simulink model "CM320A_Adc1CfgAndUse"  (R2013b)
settings: Solver=FixedStepDiscrete  SolverMode=SingleTasking  StartTime=0.0  StopTime=1  FixedStep=0.002  RelTol=1e-3
values from neighbouring files (symbols this model uses):
  ADC0CFGANDUSE_DIAGCSCANGROUPMAX_CNT_U08 = DataDict.Constant    [CM320A_Adc1CfgAndUse_DataDict.m]
  ADC0CFGANDUSE_DIAGCSCANGROUPMIN_CNT_U08 = DataDict.Constant    [CM320A_Adc1CfgAndUse_DataDict.m]
undefined symbols (not defined in the file or in its folder): sigbuilder_block
libraries: simulink x3
settings Model: Creator=nz3zln  LastModifiedBy=wzvp6q
settings SolverCC: AutoInsertRateTranBlk=on  InsertRTBMode=Always
settings DataIOCC: LimitDataPoints=off  SaveFormat=Structure  ReturnWorkspaceOutputs=on
settings OptimizationCC: BlockReduction=off  InlineParams=on  ZeroExternalMemoryAtStartup=off  ZeroInternalMemoryAtStartup=off  OptimizeModelRefInitCode=on  LifeSpan=1
settings DebuggingCC: SignalInfNanChecking=error  SignalRangeChecking=warning  UnderspecifiedInitializationDetection=Simplified  SolverPrmCheckMsg=error  DiscreteInheritContinuousMsg=error  SingleTaskRateTransMsg=error  TasksWithSamePriorityMsg=error  SigSpecEnsureSampleTimeMsg=error  CheckMatrixSingularityMsg=error  ParameterUnderflowMsg=error  ParameterPrecisionLossMsg=error  ParameterTunabilityLossMsg=error  FixptConstUnderflowMsg=warning  FixptConstOverflowMsg=warning  VectorMatrixConversionMsg=error  SignalLabelMismatchMsg=error  UnconnectedInputMsg=error  UnconnectedOutputMsg=error  UnconnectedLineMsg=error  SFcnCompatibilityMsg=error  UniqueDataStoreMsg=warning  BusObjectLabelMismatch=error  RootOutportRequireBusObject=error  AssertControl=DisableAll  ModelReferenceIOMsg=error  ModelReferenceVersionMismatchMessage=warning  ModelReferenceIOMismatchMessage=error  ModelReferenceCSMismatchMessage=warning  ModelReferenceDataLoggingMessage=error  StateNameClashWarn=warning  StrictBusMsg=ErrorOnBusTreatedAsVector  NonBusSignalsTreatedAsBus=error  SFUnexpectedBacktrackingDiag=error  SFInvalidInputDataAccessInChartInitDiag=error  SFNoUnconditionalDefaultTransitionDiag=error  SFTransitionOutsideNaturalParentDiag=error  SFUnconditionalTransitionShadowingDiag=error  SFUndirectedBroadcastEventsDiag=error
settings ModelReferenceCC: ModelReferenceNumInstancesAllowed=Single
settings RTWCC: SystemTargetFile=autosar.tlc  GenCodeOnly=on  TemplateMakefile=ert_default_tmf  Description=AUTOSAR  GenerateReport=on  ProcessScript=autosar_make_rtw_hook  LaunchReport=on
settings CodeAppCC: GenerateComments=off  IgnoreCustomStorageClasses=off  CustomSymbolStrType=$N$R$M  CustomSymbolStrBlkIO=$N$M  SimulinkBlockComments=off
settings STFCustomTargetCC: ParMdlRefBuildCompliant=on  CompOptLevelCompliant=on  IncludeMdlTerminateFcn=off  CombineOutputUpdateFcns=on  SuppressErrorStatus=on  ERTFirstTimeCompliant=on  ERTCustomFileBanners=on  SupportNonFinite=off  SupportComplex=off  SupportContinuousTime=off  SupportNonInlinedSFcns=off  MATLABClassNameForMDSCustomization=Simulink.SoftwareTarget.ERTCustomization  AutosarCompliant=on  GRTInterface=off  SystemTargetFile=autosar.tlc
settings ERTTargetCC: CodeReplacementLibrary=ANSI_C  ConcurrentExecutionCompliant=off  IncludeMdlTerminateFcn=off  SuppressErrorStatus=on  SupportNonFinite=off  SupportComplex=off  ModelStepFunctionPrototypeControlCompliant=off  CPPClassGenCompliant=off  AutosarCompliant=on  InlinedParameterPlacement=NonHierarchical  ERTCustomFileTemplate=example_file_process.tlc  EnableUserReplacementTypes=on

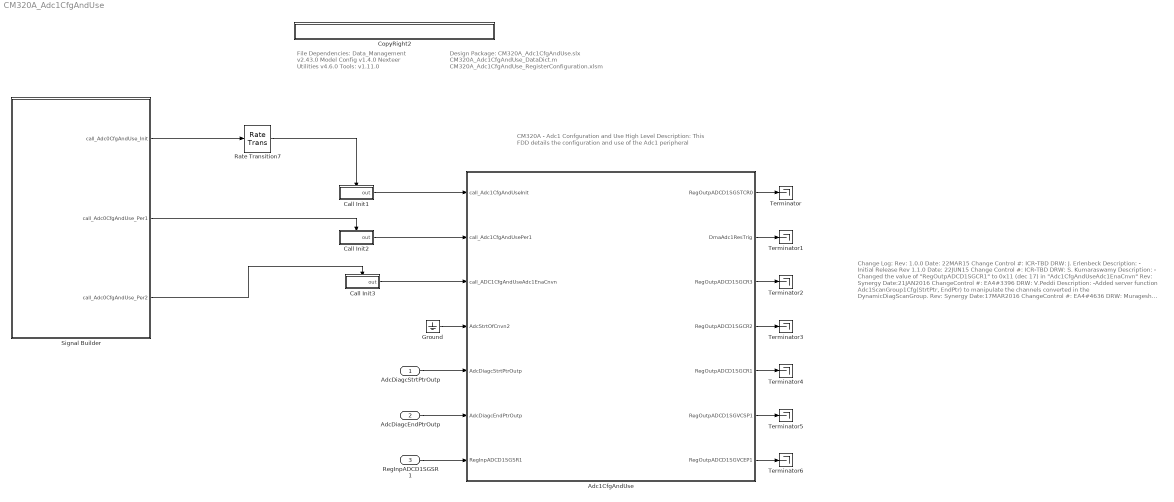
== system CM320A_Adc1CfgAndUse ==
  note: CM320A - Adc1 Confguration and Use
      |
      | High Level Description:
      | This FDD details the configuration and use of the Adc1 peripheral
  note: Change Log:
      |
      | Rev: 1.0.0
      | Date: 22MAR15
      | Change Control #: ICR-TBD
      | DRW: J. Erlenbeck
      | Description:
      | - Initial Release
      |
      | Rev 1.1.0
      | Date: 22JUN15
      | Change Control #: ICR-TBD
      | DRW: S. Kumaraswamy
      | Description:
      | - Changed the value of "RegOutpADCD1SGCR1" to 0x11 (dec 17) in "Adc1CfgAndUseAdc1EnaCnvn"
      |
      | Rev: Synergy
      | Date:21JAN2016
      | ChangeControl #: EA4#3396
      | DRW: V.Peddi
      | Description:
      | -Added server function Adc1ScanGroup1Cfg(StrtPtr, EndPtr)
      |  to manipulate the channels converted in the DynamicDiagScanGroup.
      |
      |
      | Rev: Synergy
      | Date:17MAR2016
      | ChangeControl #: EA4#4636
      | DRW: Muragesh Asundi/Lalkrishna Pandey (KPIT)
      | Description:
      | -As per anomaly CR EA4#3742, following changes are made,
      | -  Register names ADCD0SGVCEP1 and ADCD0SGVCSP1 corrected to
      | ADCD1SGVCEP1 and ADCD1SGVCSP1 respectively.
      | - All the constants and configParam properties are updated to 'Global'.
      |
      |
      | Rev 2.2.0
      | Date: 07JUN16
      | Change Control #: WCR EA4#5947
      | DRW: G. McCann
      | Description:
      | - Remove server function Adc1CfgAndUseAdc1ScanGroup1Cfg and
      |   replace with Adc1CfgAndUsePer2
      | - Make StrtPtr and EndPtr update dependent on a change in inputs and
      |   A/D converter idle state
      |
      |
      | Rev 2.3.0
      | Date: 28JUL16
      | Change Control #: WCR EA4#7446
      | DRW: G. McCann
      | Description:
      | - Initialize Adc1DiagcStrtPtr and Adc1DiagcEndPtr in Adc1CfgAndUseInit1
      | - Updated CM320A_Adc1CfgAndUse_RegisterConfiguration.xlsm to use ADCD1SGCR1 to trigger DMA
      |   instead of ADCD1SGCR3 to trigger DMA.
  note: File Dependencies:
      | Data_Management v2.43.0
      | Model Config v1.4.0
      | Nexteer Utilities v4.6.0
      | Tools: v1.11.0
  note: Design Package:
      | CM320A_Adc1CfgAndUse.slx
      | CM320A_Adc1CfgAndUse_DataDict.m
      | CM320A_Adc1CfgAndUse_RegisterConfiguration.xlsm
  AdcDiagcStrtPtrOutp : Inport
  AdcDiagcEndPtrOutp : Inport  Port=2
  RegInpADCD1SGSR1 : Inport  RequirementInfo={} %GIDa_1454e784_31d7_4f3c_b38c_eefbf3be6ffb  Port=3
  Adc1CfgAndUse : Subsystem
  Call Init1 : Subsystem  TreatAsAtomicUnit=on
  Call Init2 : Subsystem  TreatAsAtomicUnit=on
  Call Init3 : Subsystem  TreatAsAtomicUnit=on
  CopyRight2 : Subsystem  Description=|  mask(Copyright Information){none=on}
      | Copyright info block.                                               
      |                                                                     
      | Place copyright information at the top of every subsystem in design.
      mask prompts: none "No parameters"
      mask help: Place copyright information at the top of every subsystem in design.
      mask Display:
      | NxtrConf = 'Nexteer Confidential';
      | 
      | sys = bdroot; %handle for the current model ("system")
      | first = get_param(sys,'Created');
      | first = first(end-3:end);  %year is last four digits
      | 
      | last = get_param(sys,'LastModifiedDate');
      | if isempty(last)
      |     last = datestr(now,'yyyy');
      | else
      |     last = last(end-3:end);
      | end
      | 
      | if strcmp(first,last)
      |     fprintf('%s -- Copyright %s Nexteer',NxtrConf,first)
      | else
      |     fprintf('%s -- %s%s- %s Nexteer',NxtrConf,char(169),first,last)
      | end
  Ground : Ground
  Rate Transition7 : RateTransition
  Signal Builder : Subsystem  Tag=STV Subsys  RequirementInfo={} %GIDa_2822100e_29fa_4197_9ccc_01864625f252  LoadFcn=sigbuilder_block('load');  StartFcn=sigbuilder_block('start');  StopFcn=sigbuilder_block('stop');  ClipboardFcn=sigbuilder_block('clipboard');  mask(Sigbuilder block){}
      mask help: Simulink:masks:SigbuilderBlock_MD
      mask init:
      | if ~strcmp(get_param(bdroot(gcbh),'SimulationStatus'),'stopped') tuvar = sigbuilder_block('maskInit'); end
      settings: CopyFcn=sigbuilder_block('copy');  DeleteFcn=sigbuilder_block('delete');  ModelCloseFcn=sigbuilder_block('modelClose');  PreSaveFcn=sigbuilder_block('preSave');  PauseFcn=sigbuilder_block('pause');  ContinueFcn=sigbuilder_block('continue');  NameChangeFcn=sigbuilder_block('namechange');  OpenFcn=sigbuilder_block('open',[0 127.5 768 484.5 ]);  CloseFcn=sigbuilder_block('close');
      mask Display: plot(0, 0, 100, 100,[2, 2, 32, 32, 2], [68, 8, 8, 68, 68],[32, 2], [38, 38], [32, 19, 2],[53, 60, 44], [32, 17, 17, 2],[16, 16, 31, 31]);txt = getActiveGroup(gcbh);text(2, 100, txt,'verticalAlignment', 'top');
  Terminator{,1..6} (7 alike) : Terminator
  wires:
  Signal Builder/1(call_Adc0CfgAndUse_Init) -> Rate Transition7/1
  Call Init1/1(out) -> Adc1CfgAndUse/1(call_Adc1CfgAndUseInit)
  Rate Transition7/1 -> Call Init1/Enable
  Signal Builder/2(call_Adc0CfgAndUse_Per1) -> Call Init2/Enable
  Signal Builder/3(call_Adc0CfgAndUse_Per2) -> Call Init3/Enable
  Call Init2/1(out) -> Adc1CfgAndUse/2(call_Adc1CfgAndUsePer1)
  Call Init3/1(out) -> Adc1CfgAndUse/3(call_ADC1CfgAndUseAdc1EnaCnvn)
  AdcDiagcStrtPtrOutp/1 -> Adc1CfgAndUse/5(AdcDiagcStrtPtrOutp)
  AdcDiagcEndPtrOutp/1 -> Adc1CfgAndUse/6(AdcDiagcEndPtrOutp)
  RegInpADCD1SGSR1/1 -> Adc1CfgAndUse/7(RegInpADCD1SGSR1)
  Ground/1 -> Adc1CfgAndUse/4(AdcStrtOfCnvn2)
  Adc1CfgAndUse/1(RegOutpADCD1SGSTCR0) -> Terminator/1
  Adc1CfgAndUse/2(DmaAdc1ResTrig) -> Terminator1/1
  Adc1CfgAndUse/3(RegOutpADCD1SGCR3) -> Terminator2/1
  Adc1CfgAndUse/4(RegOutpADCD1SGCR2) -> Terminator3/1
  Adc1CfgAndUse/5(RegOutpADCD1SGCR1) -> Terminator4/1
  Adc1CfgAndUse/6(RegOutpADCD1SGVCSP1) -> Terminator5/1
  Adc1CfgAndUse/7(RegOutpADCD1SGVCEP1) -> Terminator6/1

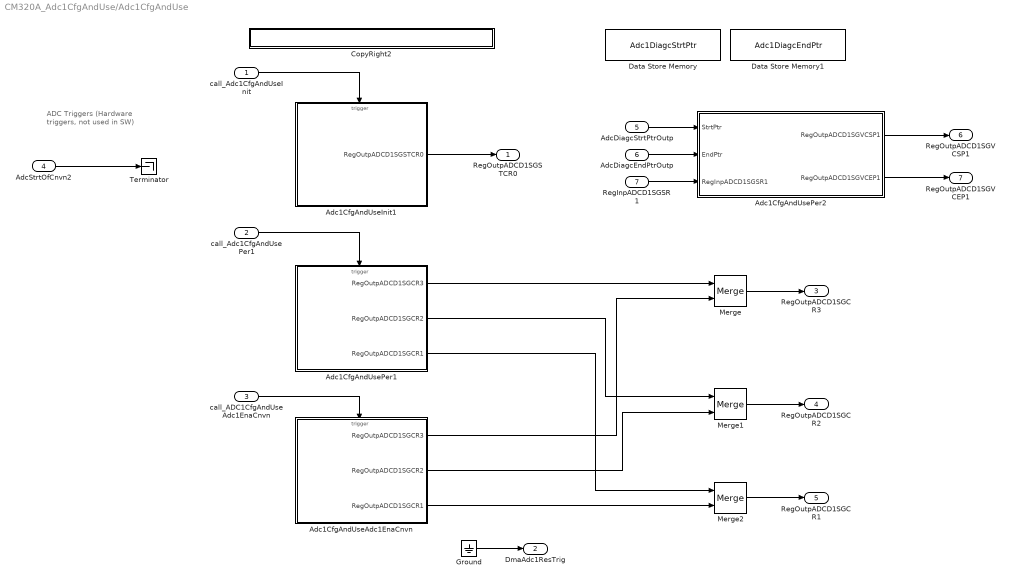
== system CM320A_Adc1CfgAndUse/Adc1CfgAndUse ==
  note: ADC Triggers
      | (Hardware triggers, not used
      | in SW)
  call_Adc1CfgAndUseInit : Inport
  call_Adc1CfgAndUsePer1 : Inport  Port=2
  call_ADC1CfgAndUseAdc1EnaCnvn : Inport  Port=3
  AdcStrtOfCnvn2 : Inport  Port=4
  AdcDiagcStrtPtrOutp : Inport  Port=5
  AdcDiagcEndPtrOutp : Inport  Port=6
  RegInpADCD1SGSR1 : Inport  RequirementInfo={} %GIDa_fca0a65f_1cb5_4b35_9a3e_e692200297bc  Port=7
  Adc1CfgAndUseAdc1EnaCnvn : Subsystem
  Adc1CfgAndUseInit1 : Subsystem
  Adc1CfgAndUsePer1 : Subsystem
  Adc1CfgAndUsePer2 : Subsystem  RequirementInfo="{'linktype_rmi_doors' '0000c475 (/ESG Group/FDD Module Requirements/EA4 Specific/CM320A_Adc1CfgAndUse)' '#CM320A_77' 'true' 'REQ:  CM320A_77' '' } %GIDa_eb0eafa5_d999_43e2_9b65_3012ac79943e"
  CopyRight2 : Subsystem  Description=|  mask(Copyright Information){none=on}
      | Copyright info block.                                               
      |                                                                     
      | Place copyright information at the top of every subsystem in design.
      mask prompts: none "No parameters"
      mask help: Place copyright information at the top of every subsystem in design.
      mask Display:
      | NxtrConf = 'Nexteer Confidential';
      | 
      | sys = bdroot; %handle for the current model ("system")
      | first = get_param(sys,'Created');
      | first = first(end-3:end);  %year is last four digits
      | 
      | last = get_param(sys,'LastModifiedDate');
      | if isempty(last)
      |     last = datestr(now,'yyyy');
      | else
      |     last = last(end-3:end);
      | end
      | 
      | if strcmp(first,last)
      |     fprintf('%s -- Copyright %s Nexteer',NxtrConf,first)
      | else
      |     fprintf('%s -- %s%s- %s Nexteer',NxtrConf,char(169),first,last)
      | end
  Data Store Memory : DataStoreMemory  DataStoreName=Adc1DiagcStrtPtr  StateMustResolveToSignalObject=on
  Data Store Memory1 : DataStoreMemory  DataStoreName=Adc1DiagcEndPtr  StateMustResolveToSignalObject=on
  Ground : Ground
  Merge : Merge
  Merge1 : Merge
  Merge2 : Merge
  Terminator : Terminator
  RegOutpADCD1SGSTCR0 : Outport  RequirementInfo={} %GIDa_38330155_36ba_489f_82a9_9da59df6df64
  DmaAdc1ResTrig : Outport  RequirementInfo={'linktype_rmi_doors' '0000c475 (/ESG Group/FDD Module Requirements/EA4 Specific/CM320A_Adc1CfgAndUse)' '#CM320A_84' 'true' 'REQ: CM320A_84' '' } %GIDa_96a67154_1cf8_4536_bab5_cb4a5a0ca20a  Port=2
  RegOutpADCD1SGCR3 : Outport  RequirementInfo={} %GIDa_36a53c96_09d9_4fd4_84b5_b5dac70e9df9  Port=3
  RegOutpADCD1SGCR2 : Outport  RequirementInfo={} %GIDa_11e2f2b9_42e8_4caf_874a_0934adb01b0a  Port=4
  RegOutpADCD1SGCR1 : Outport  RequirementInfo={} %GIDa_8357333e_8679_4d79_acb0_0ada0cf3f58e  Port=5
  RegOutpADCD1SGVCSP1 : Outport  Port=6
  RegOutpADCD1SGVCEP1 : Outport  Port=7
  wires:
  call_Adc1CfgAndUseInit/1 -> Adc1CfgAndUseInit1/Trigger
  Adc1CfgAndUseInit1/1(RegOutpADCD1SGSTCR0) -> RegOutpADCD1SGSTCR0/1
  AdcStrtOfCnvn2/1 -> Terminator/1
  Ground/1 -> DmaAdc1ResTrig/1
  call_Adc1CfgAndUsePer1/1 -> Adc1CfgAndUsePer1/Trigger
  call_ADC1CfgAndUseAdc1EnaCnvn/1 -> Adc1CfgAndUseAdc1EnaCnvn/Trigger
  Merge/1 -> RegOutpADCD1SGCR3/1
  Merge1/1 -> RegOutpADCD1SGCR2/1
  Merge2/1 -> RegOutpADCD1SGCR1/1
  Adc1CfgAndUsePer1/1(RegOutpADCD1SGCR3) -> Merge/1
  Adc1CfgAndUsePer1/2(RegOutpADCD1SGCR2) -> Merge1/1
  Adc1CfgAndUsePer1/3(RegOutpADCD1SGCR1) -> Merge2/1
  Adc1CfgAndUseAdc1EnaCnvn/1(RegOutpADCD1SGCR3) -> Merge/2
  Adc1CfgAndUseAdc1EnaCnvn/2(RegOutpADCD1SGCR2) -> Merge1/2
  Adc1CfgAndUseAdc1EnaCnvn/3(RegOutpADCD1SGCR1) -> Merge2/2
  AdcDiagcStrtPtrOutp/1 -> Adc1CfgAndUsePer2/1(StrtPtr)
  AdcDiagcEndPtrOutp/1 -> Adc1CfgAndUsePer2/2(EndPtr)
  Adc1CfgAndUsePer2/1(RegOutpADCD1SGVCSP1) -> RegOutpADCD1SGVCSP1/1
  Adc1CfgAndUsePer2/2(RegOutpADCD1SGVCEP1) -> RegOutpADCD1SGVCEP1/1
  RegInpADCD1SGSR1/1 -> Adc1CfgAndUsePer2/3(RegInpADCD1SGSR1)

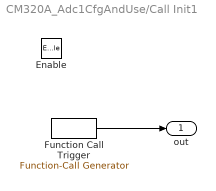
== system CM320A_Adc1CfgAndUse/Call Init1 ==
  Enable : EnablePort
  Function Call Trigger : simulink/Ports & Subsystems/Function-Call Generator  RequirementInfo="{'linktype_rmi_doors' '000089e3 (/E-STEER_New/System Specification Documents/Core Specs/Subsystem Specs/System Functions FDD/SF-46  Gross Cross Check)' '#211' 'true' '3.1-1 The GCC function shall monitor every posted output motor comm' '' ; 'linktype_rmi_doors' '000089e3 (/E-STEER_New/System Specification Documents/Core Specs/Subsystem Specs/System Functions FDD/SF-46  Gross Cross Check)' '#182' 'true' '3.2.2-1 GCC shall be executed at a 0.002 second loop time.' '' } %GIDa_ff755a2e_49d1_45f7_8591_3ce0ef475338"  sample_time=0.002  numberOfIterations=1
  out : Outport
  wires:
  Function Call Trigger/1 -> out/1

== system CM320A_Adc1CfgAndUse/Call Init2 ==
  Enable : EnablePort
  Function Call Trigger : simulink/Ports & Subsystems/Function-Call Generator  RequirementInfo="{'linktype_rmi_doors' '000089e3 (/E-STEER_New/System Specification Documents/Core Specs/Subsystem Specs/System Functions FDD/SF-46  Gross Cross Check)' '#211' 'true' '3.1-1 The GCC function shall monitor every posted output motor comm' '' ; 'linktype_rmi_doors' '000089e3 (/E-STEER_New/System Specification Documents/Core Specs/Subsystem Specs/System Functions FDD/SF-46  Gross Cross Check)' '#182' 'true' '3.2.2-1 GCC shall be executed at a 0.002 second loop time.' '' } %GIDa_d04bc59e_8291_4b90_b6fb_7973e3e96afb"  sample_time=0.002  numberOfIterations=1
  out : Outport
  wires:
  Function Call Trigger/1 -> out/1

== system CM320A_Adc1CfgAndUse/Call Init3 ==
  Enable : EnablePort
  Function Call Trigger : simulink/Ports & Subsystems/Function-Call Generator  RequirementInfo="{'linktype_rmi_doors' '000089e3 (/E-STEER_New/System Specification Documents/Core Specs/Subsystem Specs/System Functions FDD/SF-46  Gross Cross Check)' '#211' 'true' '3.1-1 The GCC function shall monitor every posted output motor comm' '' ; 'linktype_rmi_doors' '000089e3 (/E-STEER_New/System Specification Documents/Core Specs/Subsystem Specs/System Functions FDD/SF-46  Gross Cross Check)' '#182' 'true' '3.2.2-1 GCC shall be executed at a 0.002 second loop time.' '' } %GIDa_029a9e5d_cc16_4dd6_825e_fb06f1fad2b7"  sample_time=0.002  numberOfIterations=1
  out : Outport
  wires:
  Function Call Trigger/1 -> out/1

== system CM320A_Adc1CfgAndUse/CopyRight2 ==

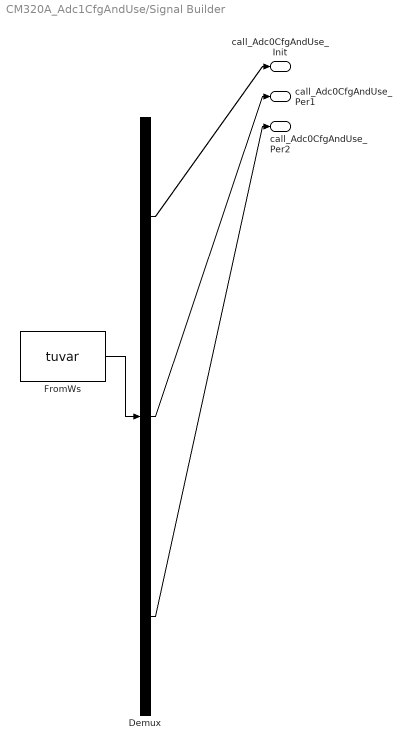
== system CM320A_Adc1CfgAndUse/Signal Builder ==
  Demux : Demux  Tag=STV Demux  Outputs=3
  FromWs : FromWorkspace  Tag=STV FromWs  VariableName=tuvar  SampleTime=0
      SigBuilderData=|
      | common.afterFinalStr = 'Extrapolate'
      | common.sampleTime = 0
      | dataSet(1).timeRange = [0 0.5]
      | dataSet(1).name = 'Group 1'
      | dataSet(2).timeRange = [0 0.5]
      | dataSet(2).name = 'Group 2'
      | dataSet(3).timeRange = [0 1.2]
      | dataSet(3).name = 'Group 3'
      | dataSet(4).timeRange = [0 5]
      | dataSet(4).name = 'Group 4'
      | dataSet(5).timeRange = [0 10]
      | dataSet(5).name = 'Group 5'
      | dataSet(6).timeRange = [0 8]
      | dataSet(6).name = 'Group 6'
      | sbobj.Groups(1).Name = 'Group 1'
      | sbobj.Groups(1).Signals(1).Name = 'call_Adc0CfgAndUse_Init'
      | sbobj.Groups(1).Signals(1).XData = [0 0.001 0.001 0.5]
      | sbobj.Groups(1).Signals(1).YData = [1 1 0 0]
      | sbobj.Groups(1).Signals(2).Name = 'call_Adc0CfgAndUse_Per1'
      | sbobj.Groups(1).Signals(2).XData = [0 0.002 0.002 0.5]
      | sbobj.Groups(1).Signals(2).YData = [0 0 1 1]
      | sbobj.Groups(1).Signals(3).Name = 'call_Adc0CfgAndUse_Per2'
      | sbobj.Groups(1).Signals(3).XData = [0 0.002 0.002 8]
      | sbobj.Groups(1).Signals(3).YData = [0 0 1 1]
      | sbobj.Groups(1).TimeRange = [0 0.5]
      | sbobj.Groups(2).Name = 'Group 2'
      | sbobj.Groups(2).Signals(1).Name = 'call_Adc0CfgAndUse_Init'
      | sbobj.Groups(2).Signals(1).XData = [0 0.001 0.001 0.5]
      | sbobj.Groups(2).Signals(1).YData = [1 1 0 0]
      | sbobj.Groups(2).Signals(2).Name = 'call_Adc0CfgAndUse_Per1'
      | sbobj.Groups(2).Signals(2).XData = [0 0.002 0.002 0.5]
      | sbobj.Groups(2).Signals(2).YData = [0 0 1 1]
      | sbobj.Groups(2).Signals(3).Name = 'call_Adc0CfgAndUse_Per2'
      | sbobj.Groups(2).Signals(3).XData = [0 0.002 0.002 8]
      | sbobj.Groups(2).Signals(3).YData = [0 0 1 1]
      | sbobj.Groups(2).TimeRange = [0 0.5]
      | sbobj.Groups(3).Name = 'Group 3'
      | sbobj.Groups(3).Signals(1).Name = 'call_Adc0CfgAndUse_Init'
      | sbobj.Groups(3).Signals(1).XData = [0 0.001 0.001 1.2]
      | sbobj.Groups(3).Signals(1).YData = [1 1 0 0]
      | sbobj.Groups(3).Signals(2).Name = 'call_Adc0CfgAndUse_Per1'
      | sbobj.Groups(3).Signals(2).XData = [0 0.002 0.002 1.2]
      | sbobj.Groups(3).Signals(2).YData = [0 0 1 1]
      | sbobj.Groups(3).Signals(3).Name = 'call_Adc0CfgAndUse_Per2'
      | sbobj.Groups(3).Signals(3).XData = [0 0.002 0.002 8]
      | sbobj.Groups(3).Signals(3).YData = [0 0 1 1]
      | sbobj.Groups(3).TimeRange = [0 1.2]
      | sbobj.Groups(4).Name = 'Group 4'
      | sbobj.Groups(4).Signals(1).Name = 'call_Adc0CfgAndUse_Init'
      | sbobj.Groups(4).Signals(1).XData = [0 0.001 0.001 5]
      | sbobj.Groups(4).Signals(1).YData = [1 1 0 0]
      | sbobj.Groups(4).Signals(2).Name = 'call_Adc0CfgAndUse_Per1'
      | sbobj.Groups(4).Signals(2).XData = [0 0.002 0.002 5]
      | sbobj.Groups(4).Signals(2).YData = [0 0 1 1]
      | sbobj.Groups(4).Signals(3).Name = 'call_Adc0CfgAndUse_Per2'
      | sbobj.Groups(4).Signals(3).XData = [0 0.002 0.002 8]
      | sbobj.Groups(4).Signals(3).YData = [0 0 1 1]
      | sbobj.Groups(4).TimeRange = [0 5]
      | sbobj.Groups(5).Name = 'Group 5'
      | sbobj.Groups(5).Signals(1).Name = 'call_Adc0CfgAndUse_Init'
      | sbobj.Groups(5).Signals(1).XData = [0 0.001 0.001 10]
      | sbobj.Groups(5).Signals(1).YData = [1 1 0 0]
      | sbobj.Groups(5).Signals(2).Name = 'call_Adc0CfgAndUse_Per1'
      | sbobj.Groups(5).Signals(2).XData = [0 0.002 0.002 10]
      | sbobj.Groups(5).Signals(2).YData = [0 0 1 1]
      | sbobj.Groups(5).Signals(3).Name = 'call_Adc0CfgAndUse_Per2'
      | sbobj.Groups(5).Signals(3).XData = [0 0.002 0.002 10]
      | sbobj.Groups(5).Signals(3).YData = [0 0 1 1]
      | sbobj.Groups(6).Name = 'Group 6'
      | sbobj.Groups(6).Signals(1).Name = 'call_Adc0CfgAndUse_Init'
      | sbobj.Groups(6).Signals(1).XData = [0 0.001 0.001 8]
      | sbobj.Groups(6).Signals(1).YData = [1 1 0 0]
      | sbobj.Groups(6).Signals(2).Name = 'call_Adc0CfgAndUse_Per1'
      | sbobj.Groups(6).Signals(2).XData = [0 0.002 0.002 8]
      | sbobj.Groups(6).Signals(2).YData = [0 0 1 1]
      | sbobj.Groups(6).Signals(3).Name = 'call_Adc0CfgAndUse_Per2'
      | sbobj.Groups(6).Signals(3).XData = [0 0.002 0.002 8]
      | sbobj.Groups(6).Signals(3).YData = [0 0 1 1]
      | sbobj.Groups(6).TimeRange = [0 8]
  call_Adc0CfgAndUse_Init : Outport  Tag=STV Outport
  call_Adc0CfgAndUse_Per1 : Outport  Tag=STV Outport  Port=2
  call_Adc0CfgAndUse_Per2 : Outport  Tag=STV Outport  Port=3
  wires:
  FromWs/1 -> Demux/1
  Demux/1 -> call_Adc0CfgAndUse_Init/1
  Demux/2 -> call_Adc0CfgAndUse_Per1/1
  Demux/3 -> call_Adc0CfgAndUse_Per2/1

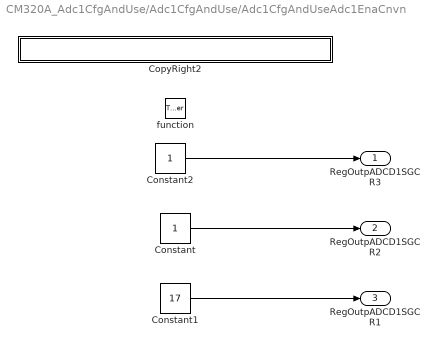
== system CM320A_Adc1CfgAndUse/Adc1CfgAndUse/Adc1CfgAndUseAdc1EnaCnvn ==
  function : TriggerPort  TriggerType=function-call
  Constant : Constant
  Constant1 : Constant  Value=17
  Constant2 : Constant
  CopyRight2 : Subsystem  Description=|  mask(Copyright Information){none=on}
      | Copyright info block.                                               
      |                                                                     
      | Place copyright information at the top of every subsystem in design.
      mask prompts: none "No parameters"
      mask help: Place copyright information at the top of every subsystem in design.
      mask Display:
      | NxtrConf = 'Nexteer Confidential';
      | 
      | sys = bdroot; %handle for the current model ("system")
      | first = get_param(sys,'Created');
      | first = first(end-3:end);  %year is last four digits
      | 
      | last = get_param(sys,'LastModifiedDate');
      | if isempty(last)
      |     last = datestr(now,'yyyy');
      | else
      |     last = last(end-3:end);
      | end
      | 
      | if strcmp(first,last)
      |     fprintf('%s -- Copyright %s Nexteer',NxtrConf,first)
      | else
      |     fprintf('%s -- %s%s- %s Nexteer',NxtrConf,char(169),first,last)
      | end
  RegOutpADCD1SGCR3 : Outport  RequirementInfo={} %GIDa_3019a61e_ffa2_47f4_8a07_737a7e5a857d
  RegOutpADCD1SGCR2 : Outport  RequirementInfo={} %GIDa_4543efc7_f62f_4a60_ba19_073d61607fbd  Port=2
  RegOutpADCD1SGCR1 : Outport  RequirementInfo={} %GIDa_f00de3c6_6335_482f_90be_12f45b9882d5  Port=3
  wires:
  Constant/1 -> RegOutpADCD1SGCR2/1
  Constant1/1 -> RegOutpADCD1SGCR1/1
  Constant2/1 -> RegOutpADCD1SGCR3/1

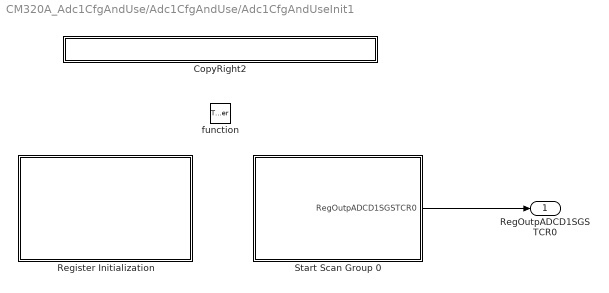
== system CM320A_Adc1CfgAndUse/Adc1CfgAndUse/Adc1CfgAndUseInit1 ==
  function : TriggerPort  TriggerType=function-call
  CopyRight2 : Subsystem  Description=|  mask(Copyright Information){none=on}
      | Copyright info block.                                               
      |                                                                     
      | Place copyright information at the top of every subsystem in design.
      mask prompts: none "No parameters"
      mask help: Place copyright information at the top of every subsystem in design.
      mask Display:
      | NxtrConf = 'Nexteer Confidential';
      | 
      | sys = bdroot; %handle for the current model ("system")
      | first = get_param(sys,'Created');
      | first = first(end-3:end);  %year is last four digits
      | 
      | last = get_param(sys,'LastModifiedDate');
      | if isempty(last)
      |     last = datestr(now,'yyyy');
      | else
      |     last = last(end-3:end);
      | end
      | 
      | if strcmp(first,last)
      |     fprintf('%s -- Copyright %s Nexteer',NxtrConf,first)
      | else
      |     fprintf('%s -- %s%s- %s Nexteer',NxtrConf,char(169),first,last)
      | end
  Register Initialization : Subsystem  Priority=10
      settings: AttributesFormatString=Priority: %<Priority>
  Start Scan Group 0 : Subsystem  RequirementInfo={'linktype_rmi_doors' '0000c475 (/ESG Group/FDD Module Requirements/EA4 Specific/CM320A_Adc1CfgAndUse)' '#CM320A_76' 'true' 'REQ: CM320A_76' '' } %GIDa_d862d82c_969a_40be_9cba_5dad28e4f649  Priority=20
      settings: AttributesFormatString=Priority: %<Priority>
  RegOutpADCD1SGSTCR0 : Outport  RequirementInfo={} %GIDa_29d6058b_2806_49c9_89f2_49c183a99fc2
  wires:
  Start Scan Group 0/1(RegOutpADCD1SGSTCR0) -> RegOutpADCD1SGSTCR0/1

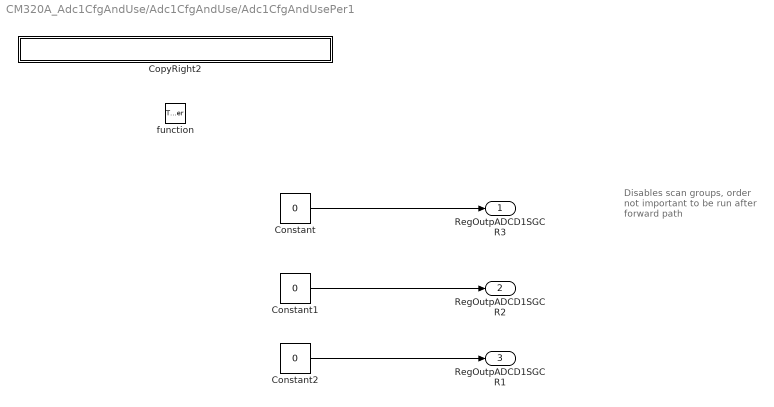
== system CM320A_Adc1CfgAndUse/Adc1CfgAndUse/Adc1CfgAndUsePer1 ==
  note: Disables scan groups,
      | order not important
      |
      | to be run after forward
      | path
  function : TriggerPort  TriggerType=function-call
  Constant : Constant  Value=0
  Constant1 : Constant  Value=0
  Constant2 : Constant  Value=0
  CopyRight2 : Subsystem  Description=|  mask(Copyright Information){none=on}
      | Copyright info block.                                               
      |                                                                     
      | Place copyright information at the top of every subsystem in design.
      mask prompts: none "No parameters"
      mask help: Place copyright information at the top of every subsystem in design.
      mask Display:
      | NxtrConf = 'Nexteer Confidential';
      | 
      | sys = bdroot; %handle for the current model ("system")
      | first = get_param(sys,'Created');
      | first = first(end-3:end);  %year is last four digits
      | 
      | last = get_param(sys,'LastModifiedDate');
      | if isempty(last)
      |     last = datestr(now,'yyyy');
      | else
      |     last = last(end-3:end);
      | end
      | 
      | if strcmp(first,last)
      |     fprintf('%s -- Copyright %s Nexteer',NxtrConf,first)
      | else
      |     fprintf('%s -- %s%s- %s Nexteer',NxtrConf,char(169),first,last)
      | end
  RegOutpADCD1SGCR3 : Outport  RequirementInfo={} %GIDa_6e095781_3705_41ec_9b48_3a2ba440ae85
  RegOutpADCD1SGCR2 : Outport  RequirementInfo={} %GIDa_5eb70d5a_e9b2_44d4_96a5_4d5692cde4c1  Port=2
  RegOutpADCD1SGCR1 : Outport  RequirementInfo={} %GIDa_9c32bcc7_998c_4584_9f76_015b71dd46e0  Port=3
  wires:
  Constant/1 -> RegOutpADCD1SGCR3/1
  Constant1/1 -> RegOutpADCD1SGCR2/1
  Constant2/1 -> RegOutpADCD1SGCR1/1

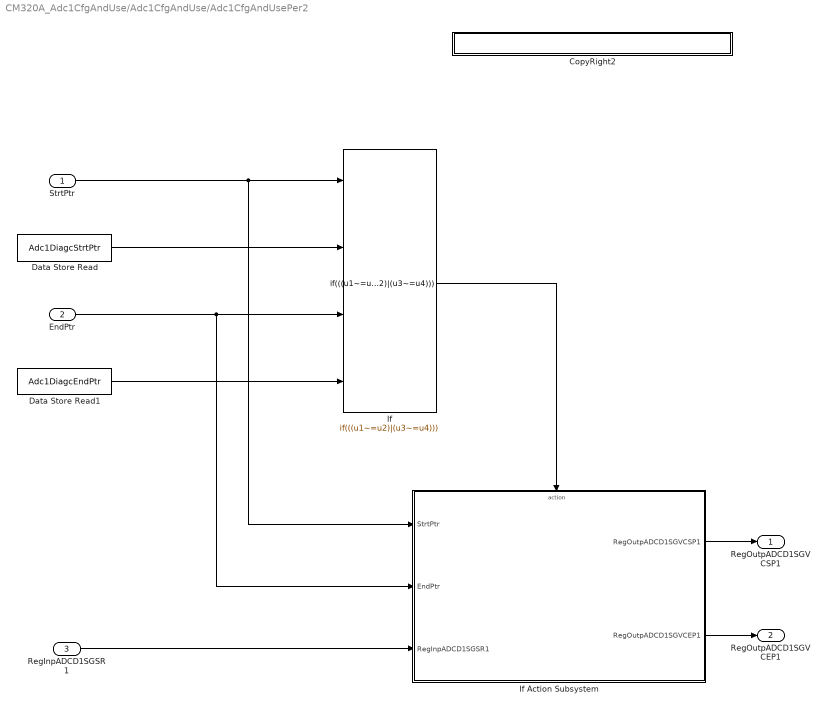
== system CM320A_Adc1CfgAndUse/Adc1CfgAndUse/Adc1CfgAndUsePer2 ==
  StrtPtr : Inport  RequirementInfo={} %GIDa_93634f1b_c019_40a7_b26a_b28bd15da65f
  EndPtr : Inport  RequirementInfo={} %GIDa_8521332f_9342_4fd9_af82_fc6809e61289  Port=2
  RegInpADCD1SGSR1 : Inport  RequirementInfo={} %GIDa_0ffd83dd_af71_495b_be08_d1c3559bc6fd  Port=3
  CopyRight2 : Subsystem  Description=|  mask(Copyright Information){none=on}
      | Copyright info block.                                               
      |                                                                     
      | Place copyright information at the top of every subsystem in design.
      mask prompts: none "No parameters"
      mask help: Place copyright information at the top of every subsystem in design.
      mask Display:
      | NxtrConf = 'Nexteer Confidential';
      | 
      | sys = bdroot; %handle for the current model ("system")
      | first = get_param(sys,'Created');
      | first = first(end-3:end);  %year is last four digits
      | 
      | last = get_param(sys,'LastModifiedDate');
      | if isempty(last)
      |     last = datestr(now,'yyyy');
      | else
      |     last = last(end-3:end);
      | end
      | 
      | if strcmp(first,last)
      |     fprintf('%s -- Copyright %s Nexteer',NxtrConf,first)
      | else
      |     fprintf('%s -- %s%s- %s Nexteer',NxtrConf,char(169),first,last)
      | end
  Data Store Read : DataStoreRead  DataStoreName=Adc1DiagcStrtPtr
  Data Store Read1 : DataStoreRead  DataStoreName=Adc1DiagcEndPtr
  If : If  NumInputs=4  IfExpression=((u1~=u2)|(u3~=u4))  ShowElse=off
  If Action Subsystem : Subsystem  TreatAsAtomicUnit=on
  RegOutpADCD1SGVCSP1 : Outport
  RegOutpADCD1SGVCEP1 : Outport  Port=2
  wires:
  StrtPtr/1 -> If Action Subsystem/1(StrtPtr), If/1
  If Action Subsystem/1(RegOutpADCD1SGVCSP1) -> RegOutpADCD1SGVCSP1/1
  If Action Subsystem/2(RegOutpADCD1SGVCEP1) -> RegOutpADCD1SGVCEP1/1
  Data Store Read/1 -> If/2
  EndPtr/1 -> If/3, If Action Subsystem/2(EndPtr)
  Data Store Read1/1 -> If/4
  If/1 -> If Action Subsystem/Action
  RegInpADCD1SGSR1/1 -> If Action Subsystem/3(RegInpADCD1SGSR1)

== system CM320A_Adc1CfgAndUse/Adc1CfgAndUse/CopyRight2 ==

== system CM320A_Adc1CfgAndUse/Adc1CfgAndUse/Adc1CfgAndUseAdc1EnaCnvn/CopyRight2 ==

== system CM320A_Adc1CfgAndUse/Adc1CfgAndUse/Adc1CfgAndUseInit1/CopyRight2 ==

== system CM320A_Adc1CfgAndUse/Adc1CfgAndUse/Adc1CfgAndUseInit1/Register Initialization ==
  note: Adc1 Configuration
      | Initialize the Adc1 registers from the following sources in the order listed:
      |
      | 1. CM320A_Adc1CfgAndUse_RegisterConfiguration.xlsm
      |     Order by row - up to Read only Registers
  CopyRight2 : Subsystem  Description=|  mask(Copyright Information){none=on}
      | Copyright info block.                                               
      |                                                                     
      | Place copyright information at the top of every subsystem in design.
      mask prompts: none "No parameters"
      mask help: Place copyright information at the top of every subsystem in design.
      mask Display:
      | NxtrConf = 'Nexteer Confidential';
      | 
      | sys = bdroot; %handle for the current model ("system")
      | first = get_param(sys,'Created');
      | first = first(end-3:end);  %year is last four digits
      | 
      | last = get_param(sys,'LastModifiedDate');
      | if isempty(last)
      |     last = datestr(now,'yyyy');
      | else
      |     last = last(end-3:end);
      | end
      | 
      | if strcmp(first,last)
      |     fprintf('%s -- Copyright %s Nexteer',NxtrConf,first)
      | else
      |     fprintf('%s -- %s%s- %s Nexteer',NxtrConf,char(169),first,last)
      | end

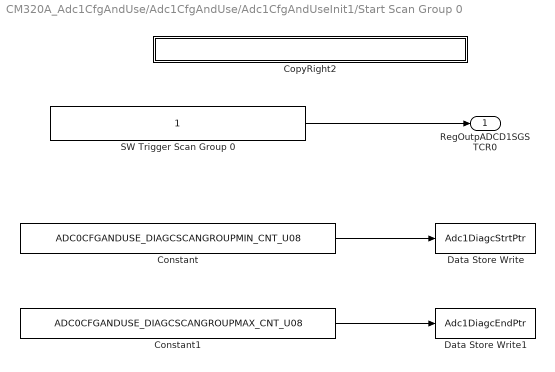
== system CM320A_Adc1CfgAndUse/Adc1CfgAndUse/Adc1CfgAndUseInit1/Start Scan Group 0 ==
  Constant : Constant  Value=ADC0CFGANDUSE_DIAGCSCANGROUPMIN_CNT_U08
  Constant1 : Constant  Value=ADC0CFGANDUSE_DIAGCSCANGROUPMAX_CNT_U08
  CopyRight2 : Subsystem  Description=|  mask(Copyright Information){none=on}
      | Copyright info block.                                               
      |                                                                     
      | Place copyright information at the top of every subsystem in design.
      mask prompts: none "No parameters"
      mask help: Place copyright information at the top of every subsystem in design.
      mask Display:
      | NxtrConf = 'Nexteer Confidential';
      | 
      | sys = bdroot; %handle for the current model ("system")
      | first = get_param(sys,'Created');
      | first = first(end-3:end);  %year is last four digits
      | 
      | last = get_param(sys,'LastModifiedDate');
      | if isempty(last)
      |     last = datestr(now,'yyyy');
      | else
      |     last = last(end-3:end);
      | end
      | 
      | if strcmp(first,last)
      |     fprintf('%s -- Copyright %s Nexteer',NxtrConf,first)
      | else
      |     fprintf('%s -- %s%s- %s Nexteer',NxtrConf,char(169),first,last)
      | end
  Data Store Write : DataStoreWrite  DataStoreName=Adc1DiagcStrtPtr
  Data Store Write1 : DataStoreWrite  DataStoreName=Adc1DiagcEndPtr
  SW Trigger Scan Group 0 : Constant  OutDataTypeStr=uint32
  RegOutpADCD1SGSTCR0 : Outport  RequirementInfo={} %GIDa_c6fe82bc_6768_4bbb_8f71_a05cf9df8531
  wires:
  SW Trigger Scan Group 0/1 -> RegOutpADCD1SGSTCR0/1
  Constant/1 -> Data Store Write/1
  Constant1/1 -> Data Store Write1/1

== system CM320A_Adc1CfgAndUse/Adc1CfgAndUse/Adc1CfgAndUsePer1/CopyRight2 ==

== system CM320A_Adc1CfgAndUse/Adc1CfgAndUse/Adc1CfgAndUsePer2/CopyRight2 ==

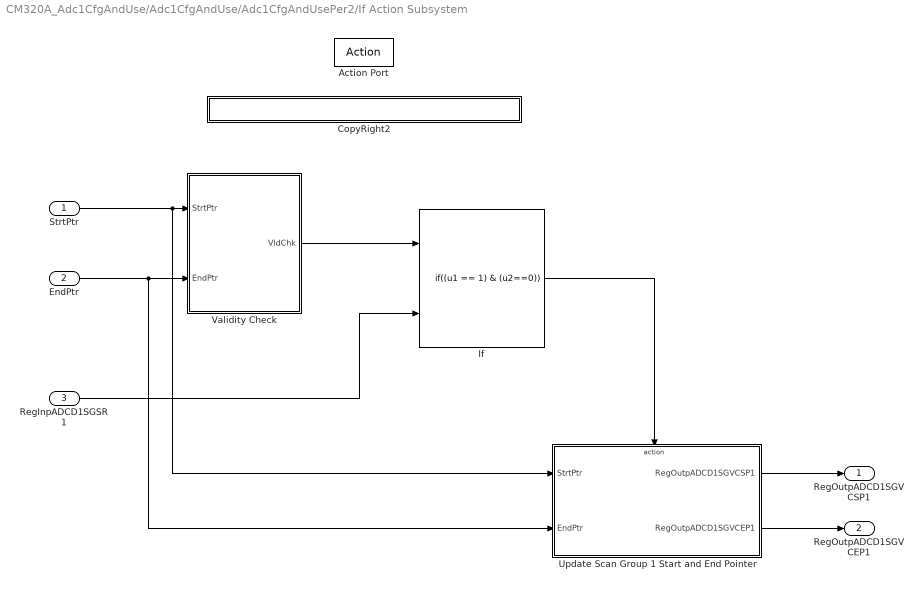
== system CM320A_Adc1CfgAndUse/Adc1CfgAndUse/Adc1CfgAndUsePer2/If Action Subsystem ==
  StrtPtr : Inport  RequirementInfo={} %GIDa_c2a2cd30_0ad4_4db0_afb9_3b99ca9f7076
  EndPtr : Inport  RequirementInfo={} %GIDa_20023ace_af7b_481d_8509_bb21aefd96ba  Port=2
  RegInpADCD1SGSR1 : Inport  RequirementInfo={} %GIDa_0618ad18_9cd6_495f_83b5_35ef9ef73099  Port=3
  Action Port : ActionPort  ActionType=then
  CopyRight2 : Subsystem  Description=|  mask(Copyright Information){none=on}
      | Copyright info block.                                               
      |                                                                     
      | Place copyright information at the top of every subsystem in design.
      mask prompts: none "No parameters"
      mask help: Place copyright information at the top of every subsystem in design.
      mask Display:
      | NxtrConf = 'Nexteer Confidential';
      | 
      | sys = bdroot; %handle for the current model ("system")
      | first = get_param(sys,'Created');
      | first = first(end-3:end);  %year is last four digits
      | 
      | last = get_param(sys,'LastModifiedDate');
      | if isempty(last)
      |     last = datestr(now,'yyyy');
      | else
      |     last = last(end-3:end);
      | end
      | 
      | if strcmp(first,last)
      |     fprintf('%s -- Copyright %s Nexteer',NxtrConf,first)
      | else
      |     fprintf('%s -- %s%s- %s Nexteer',NxtrConf,char(169),first,last)
      | end
  If : If  NumInputs=2  IfExpression=(u1 == 1) & (u2==0)  ShowElse=off
  Update Scan Group 1 Start and End Pointer : Subsystem  RequirementInfo="{'linktype_rmi_doors' '0000c475 (/ESG Group/FDD Module Requirements/EA4 Specific/CM320A_Adc1CfgAndUse)' '#CM320A_93' 'true' 'REQ:  CM320A_93' '' } %GIDa_a8c15032_0418_4ac0_8ff8_b838088903bc"  TreatAsAtomicUnit=on
  Validity Check : Subsystem  RequirementInfo="{'linktype_rmi_doors' '0000c475 (/ESG Group/FDD Module Requirements/EA4 Specific/CM320A_Adc1CfgAndUse)' '#CM320A_75' 'true' 'REQ:  CM320A_75' '' } %GIDa_7927e88f_47b6_4858_b7a6_e79393362f2c"
  RegOutpADCD1SGVCSP1 : Outport
  RegOutpADCD1SGVCEP1 : Outport  Port=2
  wires:
  If/1 -> Update Scan Group 1 Start and End Pointer/Action
  Update Scan Group 1 Start and End Pointer/1(RegOutpADCD1SGVCSP1) -> RegOutpADCD1SGVCSP1/1
  Update Scan Group 1 Start and End Pointer/2(RegOutpADCD1SGVCEP1) -> RegOutpADCD1SGVCEP1/1
  StrtPtr/1 -> Update Scan Group 1 Start and End Pointer/1(StrtPtr), Validity Check/1(StrtPtr)
  EndPtr/1 -> Update Scan Group 1 Start and End Pointer/2(EndPtr), Validity Check/2(EndPtr)
  Validity Check/1(VldChk) -> If/1
  RegInpADCD1SGSR1/1 -> If/2

== system CM320A_Adc1CfgAndUse/Adc1CfgAndUse/Adc1CfgAndUseInit1/Register Initialization/CopyRight2 ==

== system CM320A_Adc1CfgAndUse/Adc1CfgAndUse/Adc1CfgAndUseInit1/Start Scan Group 0/CopyRight2 ==

== system CM320A_Adc1CfgAndUse/Adc1CfgAndUse/Adc1CfgAndUsePer2/If Action Subsystem/CopyRight2 ==

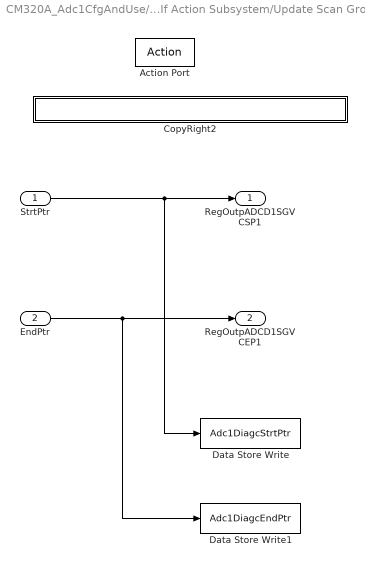
== system CM320A_Adc1CfgAndUse/Adc1CfgAndUse/Adc1CfgAndUsePer2/If Action Subsystem/Update Scan Group 1 Start and End Pointer ==
  StrtPtr : Inport
  EndPtr : Inport  Port=2
  Action Port : ActionPort  ActionType=then
  CopyRight2 : Subsystem  Description=|  mask(Copyright Information){none=on}
      | Copyright info block.                                               
      |                                                                     
      | Place copyright information at the top of every subsystem in design.
      mask prompts: none "No parameters"
      mask help: Place copyright information at the top of every subsystem in design.
      mask Display:
      | NxtrConf = 'Nexteer Confidential';
      | 
      | sys = bdroot; %handle for the current model ("system")
      | first = get_param(sys,'Created');
      | first = first(end-3:end);  %year is last four digits
      | 
      | last = get_param(sys,'LastModifiedDate');
      | if isempty(last)
      |     last = datestr(now,'yyyy');
      | else
      |     last = last(end-3:end);
      | end
      | 
      | if strcmp(first,last)
      |     fprintf('%s -- Copyright %s Nexteer',NxtrConf,first)
      | else
      |     fprintf('%s -- %s%s- %s Nexteer',NxtrConf,char(169),first,last)
      | end
  Data Store Write : DataStoreWrite  DataStoreName=Adc1DiagcStrtPtr
  Data Store Write1 : DataStoreWrite  DataStoreName=Adc1DiagcEndPtr
  RegOutpADCD1SGVCSP1 : Outport
  RegOutpADCD1SGVCEP1 : Outport  Port=2
  wires:
  StrtPtr/1 -> Data Store Write/1, RegOutpADCD1SGVCSP1/1
  EndPtr/1 -> Data Store Write1/1, RegOutpADCD1SGVCEP1/1

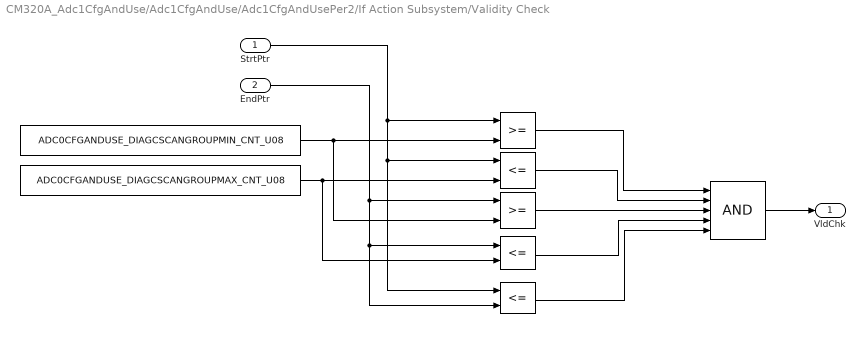
== system CM320A_Adc1CfgAndUse/Adc1CfgAndUse/Adc1CfgAndUsePer2/If Action Subsystem/Validity Check ==
  StrtPtr : Inport  RequirementInfo={} %GIDa_b61e0e57_6431_4976_be29_f5bcd7910c51
  EndPtr : Inport  RequirementInfo={} %GIDa_44d9dd4c_9956_4c45_bdfc_8f9ee083301c  Port=2
  " " : Constant  RequirementInfo={} %GIDa_b78bbcf6_7d9c_412e_a107_e54587470d06  Value=ADC0CFGANDUSE_DIAGCSCANGROUPMIN_CNT_U08
  "  " : RelationalOperator  RequirementInfo={} %GIDa_effcf520_0b3b_445a_afbd_d9aa12bbcc2f  OutDataTypeStr=boolean
  "   " : Constant  RequirementInfo={} %GIDa_1625190d_6af7_466a_830a_11acfd76d467  Value=ADC0CFGANDUSE_DIAGCSCANGROUPMAX_CNT_U08
  "     " : RelationalOperator  RequirementInfo={} %GIDa_bbd15d06_f445_44c6_84bb_8e164b4e9b04  Operator=<=  OutDataTypeStr=boolean
  "      " : RelationalOperator  RequirementInfo={} %GIDa_3ffbfb84_9708_47b6_94aa_92b9b526b7ef  Operator=<=  OutDataTypeStr=boolean
  "       " : RelationalOperator  RequirementInfo={} %GIDa_94151ad0_2a45_4614_97ff_02c06216d4e5  OutDataTypeStr=boolean
  "         " : RelationalOperator  RequirementInfo={} %GIDa_cfb8a6bc_ad67_4fd6_8bbf_49d73c54fa78  Operator=<=  OutDataTypeStr=boolean
  "          " : Logic  RequirementInfo={} %GIDa_b868517d_24e3_4483_8017_6b53ab90ffa3  Inputs=5  AllPortsSameDT=off  OutDataTypeStr=boolean
  VldChk : Outport
  wires:
  "         "/1 -> "          "/2
  EndPtr/1 -> "      "/2, "     "/1, "       "/1
  "   "/1 -> "     "/2, "         "/2
  StrtPtr/1 -> "      "/1, "         "/1, "  "/1
  "     "/1 -> "          "/4
  "          "/1 -> VldChk/1
  "       "/1 -> "          "/3
  " "/1 -> "       "/2, "  "/2
  "      "/1 -> "          "/5
  "  "/1 -> "          "/1

== system CM320A_Adc1CfgAndUse/Adc1CfgAndUse/Adc1CfgAndUsePer2/If Action Subsystem/Update Scan Group 1 Start and End Pointer/CopyRight2 ==
